simulink model "LunarLander"  (R2020a)
settings: Solver=VariableStepAuto  StartTime=0.0  StopTime=33  RelTol=1e-3
settings Model: Creator=BEAR  LastModifiedBy=bzhan
settings DataIOCC: ReturnWorkspaceOutputs=off
settings DebuggingCC: ArithmeticOperatorsInVariantConditions=warning
settings SFSimCC: SimUseLocalCustomCode=off  CustomCodeUndefinedFunction=UseInterfaceOnly
settings RTWCC: RTWUseLocalCustomCode=off

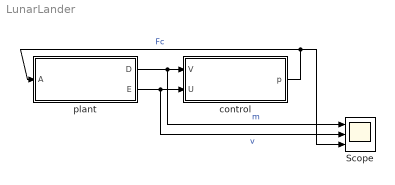
== system LunarLander ==
  Scope : Scope  NumInputPorts=3
  control : Subsystem
  plant : Subsystem
  wires:
  control/1(p) -> plant/1(A), Scope/3  "Fc"
  plant/2(E) -> Scope/2, control/2(U)  "v"
  plant/1(D) -> Scope/1, control/1(V)  "m"

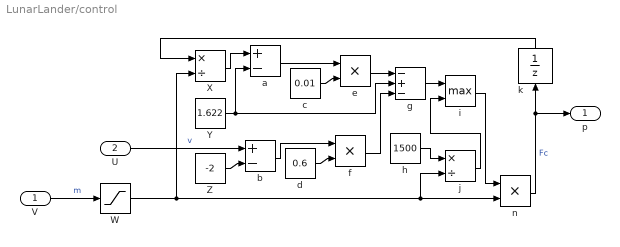
== system LunarLander/control ==
  V : Inport
  U : Inport  Port=2
  W : Saturate  UpperLimit=5000  LowerLimit=1500
  X : Product  Inputs=*/  SampleTime=0.128
  Y : Constant  Value=1.622
  Z : Constant  Value=-2
  a : Sum  Inputs=+-  SampleTime=0.128
  b : Sum  Inputs=+-  SampleTime=0.128
  c : Constant  Value=0.01
  d : Constant  Value=0.6
  e : Product  Inputs=**  SampleTime=0.128
  f : Product  Inputs=**  SampleTime=0.128
  g : Sum  Inputs=-+-  SampleTime=0.128
  h : Constant  Value=1500
  i : MinMax  Function=max  Inputs=2  SampleTime=0.128
  j : Product  Inputs=*/  SampleTime=0.128
  k : UnitDelay  InitialCondition=2027.5  SampleTime=0.128  HasFrameUpgradeWarning=on
  n : Product  Inputs=**  SampleTime=0.128
  p : Outport  VectorParamsAs1DForOutWhenUnconnected=off
  wires:
  X/1 -> a/1
  Y/1 -> g/2, a/2
  a/1 -> e/1
  c/1 -> e/2
  Z/1 -> b/2
  b/1 -> f/1
  d/1 -> f/2
  f/1 -> g/3
  U/1 -> b/1  "v"
  g/1 -> i/1
  k/1 -> X/1
  e/1 -> g/1
  W/1 -> n/2, j/2, X/2
  n/1 -> k/1, p/1  "Fc"
  i/1 -> n/1
  h/1 -> j/1
  j/1 -> i/2
  V/1 -> W/1  "m"

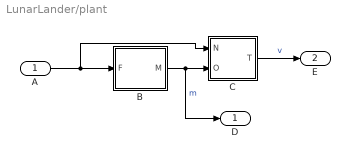
== system LunarLander/plant ==
  A : Inport
  B : Subsystem
  C : Subsystem
  D : Outport  VectorParamsAs1DForOutWhenUnconnected=off
  E : Outport  Port=2  VectorParamsAs1DForOutWhenUnconnected=off
  wires:
  B/1(M) -> C/2(O), D/1  "m"
  C/1(T) -> E/1  "v"
  A/1 -> C/1(N), B/1(F)

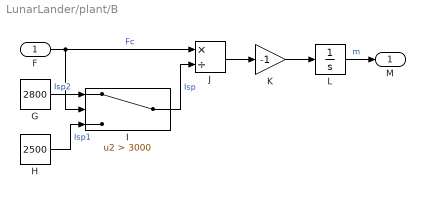
== system LunarLander/plant/B ==
  F : Inport
  G : Constant  Value=2800
  H : Constant  Value=2500
  I : Switch  Criteria=u2 > Threshold  Threshold=3000
  J : Product  Inputs=*/
  K : Gain  Gain=-1
  L : Integrator  InitialCondition=1250
  M : Outport  VectorParamsAs1DForOutWhenUnconnected=off
  wires:
  F/1 -> J/1, I/2  "Fc"
  J/1 -> K/1
  K/1 -> L/1
  L/1 -> M/1  "m"
  G/1 -> I/1  "Isp2"
  H/1 -> I/3  "Isp1"
  I/1 -> J/2  "Isp"

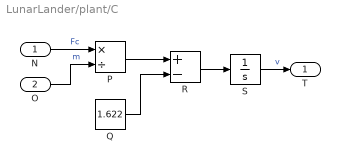
== system LunarLander/plant/C ==
  N : Inport
  O : Inport  Port=2
  P : Product  Inputs=*/
  Q : Constant  Value=1.622
  R : Sum  Inputs=+-
  S : Integrator  InitialCondition=-2
  T : Outport  VectorParamsAs1DForOutWhenUnconnected=off
  wires:
  N/1 -> P/1  "Fc"
  O/1 -> P/2  "m"
  P/1 -> R/1
  Q/1 -> R/2
  R/1 -> S/1
  S/1 -> T/1  "v"
